simulink model "test"  (R2024b)
settings: Solver=VariableStepAuto  StartTime=0.0  StopTime=10.0  RelTol=1e-3
settings Model: Creator=tsvetan  LastModifiedBy=tsvetan

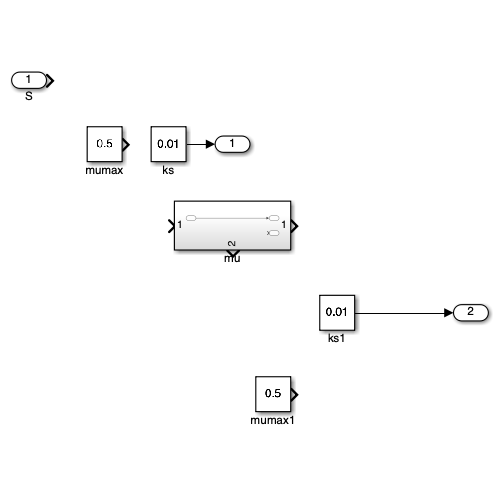
[thumbnail: Simulink's stored preview of the top-level diagram]
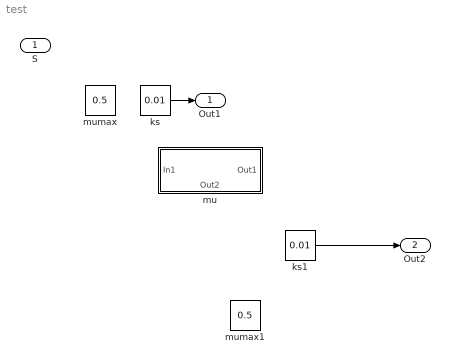
== system test ==
  S : Inport
  ks : Constant  Value=0.01
  ks1 : Constant  Value=0.01
  mu : Subsystem
      settings: PortSchema="{\"entries\":[{\"content\":{\"sides\":[{\"content\":{\"connectorIds\":[\"In1\"]},\"type\":\"ConnectorPlacement.EquallySpacedRectSide\",\"uuid\":\"a6e635a6-4007-4649-a7b8-484abb7415bc\"},{\"content\":{\"connectorIds\":[\"Out1\"],\"side\":\"RIGHT\"},\"type\":\"ConnectorPlacement.EquallySpacedRectSide\",\"uuid\":\"eb4236f6-827d-4522-b902-ca2b49a9f882\"},{\"content\":{\"side\":\"TOP\"},\"type\":\"ConnectorPlacement.EquallySpacedRectSide\",\"uuid\":\"eb41a33c-2e37-453c-a771-2473797659ad\"},{\"content\":{\"connectorIds\":[\"Out2\"],\"side\":\"BOTTOM\"},\"type\":\"ConnectorPlacement.EquallySpacedRectSide\",\"uuid\":\"9a5860a4-107f-42fc-b12e-5d5a1df0e8c6\"}]},\"type\":\"ConnectorPlacement.EquallySpacedConnector\",\"uuid\":\"bcbfa591-393a-41e2-8433-a485cf0ce821\"}],\"packageUris\":[\"http://schema.mathworks.com/mf0/Connector/R2020b\"],\"version\":\"1.0\"}"
  mumax : Constant  Value=0.5
  mumax1 : Constant  Value=0.5
  Out1 : Outport
  Out2 : Outport  Port=2
  wires:
  ks/1 -> Out1/1
  ks1/1 -> Out2/1

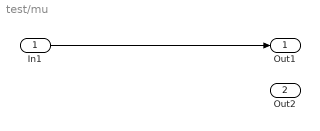
== system test/mu ==
  In1 : Inport
  Out1 : Outport
  Out2 : Outport  Port=2
  wires:
  In1/1 -> Out1/1
